simulink model "ES106A_StHlthSigStc"  (R2013b)
settings: Solver=FixedStepDiscrete  SolverMode=SingleTasking  StartTime=0.0  StopTime=1  FixedStep=0.002  RelTol=1e-3
values from neighbouring files (symbols this model uses):
  APPL10_CNT_U08 = DataDict.Constant    [ES106A_StHlthSigStc_DataDict.m]
  BITSPERBYTE_CNT_U08 = DataDict.Constant    [ES106A_StHlthSigStc_DataDict.m]
  ENOTOK_CNT_U08 = DataDict.Constant    [ES106A_StHlthSigStc_DataDict.m]
  EOK_CNT_U08 = DataDict.Constant    [ES106A_StHlthSigStc_DataDict.m]
  LOWRMASKVAL_CNT_U32 = DataDict.Constant    [ES106A_StHlthSigStc_DataDict.m]
  NROFCRCAREA_CNT_U08 = DataDict.ConfigParam    [ES106A_StHlthSigStc_DataDict.m]
  NVMAVRGPOSN_CNT_U08 = DataDict.Constant    [ES106A_StHlthSigStc_DataDict.m]
  NVMMAXPOSN_CNT_U08 = DataDict.Constant    [ES106A_StHlthSigStc_DataDict.m]
  NVMMINPOSN_CNT_U08 = DataDict.Constant    [ES106A_StHlthSigStc_DataDict.m]
  NVMSAMPLECNTRPOSN_CNT_U08 = DataDict.Constant    [ES106A_StHlthSigStc_DataDict.m]
  RAMAVRGPOSN_CNT_U08 = DataDict.Constant    [ES106A_StHlthSigStc_DataDict.m]
  RAMMAXPOSN_CNT_U08 = DataDict.Constant    [ES106A_StHlthSigStc_DataDict.m]
  RAMMINPOSN_CNT_U08 = DataDict.Constant    [ES106A_StHlthSigStc_DataDict.m]
  RAMRAWPOSN_CNT_U08 = DataDict.Constant    [ES106A_StHlthSigStc_DataDict.m]
  SIGCNT_ULS_U08 = DataDict.ConfigParam    [ES106A_StHlthSigStc_DataDict.m]
  SigStcPrmInst = DataDict.PIM    [ES106A_StHlthSigStc_DataDict.m]
  STHLTHMAXVAL_CNT_U08 = DataDict.Constant    [ES106A_StHlthSigStc_DataDict.m]
  WORDSIZE_CNT_U08 = DataDict.Constant    [ES106A_StHlthSigStc_DataDict.m]
undefined symbols (not defined in the file or in its folder): NvmGetErrSts1, StHlthTaskRef1
libraries: simulink x37, NxtrNvM x4, NxtrMax x4, NxtrMin x4
(part 1 of 5)
settings Model: Creator=SumitG  LastModifiedBy=BZHF94
settings SolverCC: AutoInsertRateTranBlk=on  InsertRTBMode=Always
settings DataIOCC: LimitDataPoints=off  SaveFormat=Structure  ReturnWorkspaceOutputs=on
settings OptimizationCC: BlockReduction=off  InlineParams=on  ZeroExternalMemoryAtStartup=off  ZeroInternalMemoryAtStartup=off  OptimizeModelRefInitCode=on  LifeSpan=1
settings DebuggingCC: SignalInfNanChecking=error  SignalRangeChecking=warning  UnderspecifiedInitializationDetection=Simplified  SolverPrmCheckMsg=error  InheritedTsInSrcMsg=error  DiscreteInheritContinuousMsg=error  SingleTaskRateTransMsg=error  TasksWithSamePriorityMsg=error  SigSpecEnsureSampleTimeMsg=error  CheckMatrixSingularityMsg=error  ParameterUnderflowMsg=error  ParameterPrecisionLossMsg=error  ParameterTunabilityLossMsg=error  FixptConstUnderflowMsg=warning  FixptConstOverflowMsg=warning  VectorMatrixConversionMsg=error  SignalLabelMismatchMsg=error  UnconnectedInputMsg=error  UnconnectedOutputMsg=error  UnconnectedLineMsg=error  SFcnCompatibilityMsg=error  UniqueDataStoreMsg=warning  BusObjectLabelMismatch=error  RootOutportRequireBusObject=error  AssertControl=DisableAll  ModelReferenceIOMsg=error  ModelReferenceVersionMismatchMessage=warning  ModelReferenceIOMismatchMessage=error  ModelReferenceCSMismatchMessage=warning  ModelReferenceDataLoggingMessage=error  StateNameClashWarn=warning  StrictBusMsg=ErrorOnBusTreatedAsVector  NonBusSignalsTreatedAsBus=error  SFUnexpectedBacktrackingDiag=error  SFInvalidInputDataAccessInChartInitDiag=error  SFNoUnconditionalDefaultTransitionDiag=error  SFTransitionOutsideNaturalParentDiag=error  SFUnconditionalTransitionShadowingDiag=error  SFUndirectedBroadcastEventsDiag=error
settings ModelReferenceCC: ModelReferenceNumInstancesAllowed=Single
settings RTWCC: SystemTargetFile=autosar.tlc  GenCodeOnly=on  TemplateMakefile=ert_default_tmf  Description=AUTOSAR  GenerateReport=on  ProcessScript=autosar_make_rtw_hook  LaunchReport=on
settings CodeAppCC: GenerateComments=off  IgnoreCustomStorageClasses=off  CustomSymbolStrType=$N$R$M  CustomSymbolStrBlkIO=$N$M  SimulinkBlockComments=off
settings STFCustomTargetCC: ParMdlRefBuildCompliant=on  CompOptLevelCompliant=on  IncludeMdlTerminateFcn=off  CombineOutputUpdateFcns=on  SuppressErrorStatus=on  ERTFirstTimeCompliant=on  ERTCustomFileBanners=on  SupportNonFinite=off  SupportComplex=off  SupportContinuousTime=off  SupportNonInlinedSFcns=off  MATLABClassNameForMDSCustomization=Simulink.SoftwareTarget.ERTCustomization  AutosarCompliant=on  GRTInterface=off  SystemTargetFile=autosar.tlc
settings ERTTargetCC: CodeReplacementLibrary=ANSI_C  ConcurrentExecutionCompliant=off  IncludeMdlTerminateFcn=off  SuppressErrorStatus=on  SupportNonFinite=off  SupportComplex=off  ModelStepFunctionPrototypeControlCompliant=off  CPPClassGenCompliant=off  AutosarCompliant=on  InlinedParameterPlacement=NonHierarchical  ERTCustomFileTemplate=example_file_process.tlc  EnableUserReplacementTypes=on

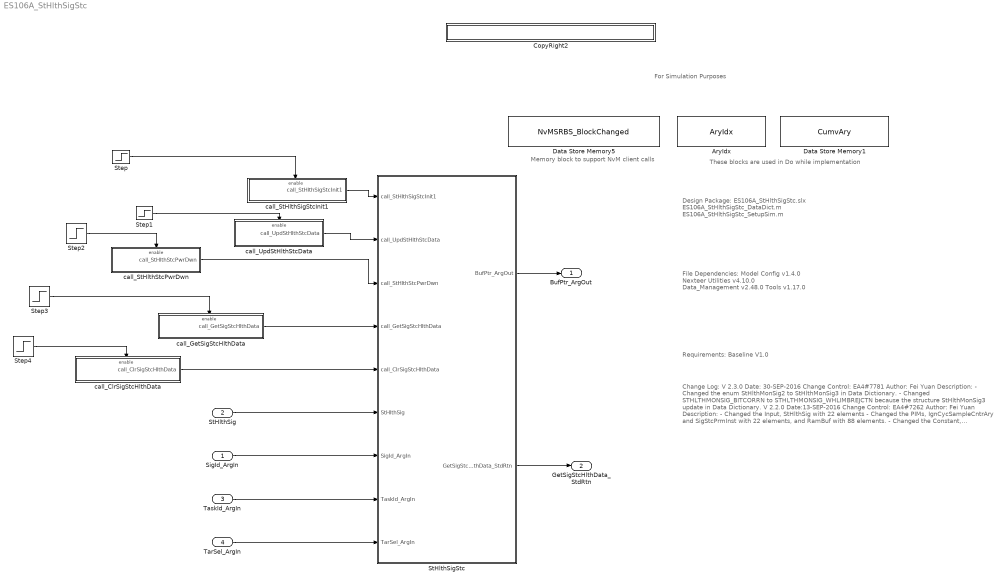
== system ES106A_StHlthSigStc ==
  note: These blocks are used in Do while implementation
  note: For Simulation Purposes
  note: Memory block to support NvM client calls
  note: Requirements: Baseline V1.0
  note: File Dependencies:
      |
      | Model Config v1.4.0
      | Nexteer Utilities v4.10.0
      | Data_Management v2.48.0
      | Tools v1.17.0
  note: Change Log:
      |
      | V 2.3.0
      | Date: 30-SEP-2016
      | Change Control: EA4#7781
      | Author: Fei Yuan
      | Description:
      | - Changed the enum StHlthMonSig2 to StHlthMonSig3 in Data Dictionary.
      | - Changed STHLTHMONSIG_BITCORRN to STHLTHMONSIG_WHLIMBREJCTN because the structure StHlthMonSig3 update in
      |   Data Dictionary.
      |
      | V 2.2.0
      | Date:13-SEP-2016
      | Change Control: EA4#7262
      | Author: Fei Yuan
      | Description:
      | - Changed the Input, StHlthSig with 22 elements
      | - Changed the PIMs, IgnCycSampleCntrAry and SigStcPrmInst with 22 elements, and RamBuf with 88 elements.
      | - Changed the Constant, SIGCNT_ULS_U08.EngVal to 22.
      | - Changed the input port size of the selectors in the model in red.
      |
      | V 2.1.0
      | Date: 2-MAY-2016
      | Change Control:  EA4#5551
      | Author: Sumit Kumar Gupta (KPIT)
      | Description:
      | - Logic added to handle 20 input signals at following subystems:
      | ES106A_StHlthSigStc/StHlthSigStc/StHlthSigStcInit1/For Simulation Purpose
      | ES106A_StHlthSigStc/StHlthSigStc/ClrSigStcHlthData/ClrDataSample/For Iterator Subsystem
      | ES106A_StHlthSigStc/StHlthSigStc/ClrSigStcHlthData/Call Non Trusted Function/For Iterator Subsystem
      |
      | - Due to MIL failures, Ram Buffer and Signal Statistic History Data Array logic is updated at following path:
      | ES106A_StHlthSigStc/StHlthSigStc/UpdStHlthStcData/UpdDataSample/For Iterator Subsystem/Subsystem2/UpdateRamBuf
      | ES106A_StHlthSigStc/StHlthSigStc/UpdStHlthStcData/Call Non Trusted Function /For Iterator Subsystem/Subsystem2/UpdateRamBuf
      | ES106A_StHlthSigStc/StHlthSigStc/StHlthStcPwrDwn/For Iterator Subsystem/If Action Subsystem/Update Nvm
      |
      | V 2.0.0
      | Date: 27-APR-2016
      | Change Control # EA4#5551
      | Author: Sumit Kumar Gupta (KPIT)
      | Description:
      | - Made the changes suggested during MIL and
      | - Changed the design to have 20 input signals coming from ES105A
      |
      | V 1.0.0
      | Date: 11-Feb-2016
      | Change Control # EA4#3078
      | Author: Sumit Kumar Gupta (KPIT)
      | Description:
      | - Initial Release
  note: Design Package:
      |
      | ES106A_StHlthSigStc.slx
      | ES106A_StHlthSigStc_DataDict.m
      | ES106A_StHlthSigStc_SetupSim.m
  SigId_ArgIn : Inport
  StHlthSig : Inport  Port=2  PortDimensions=22
  TaskId_ArgIn : Inport  Port=3
  TarSel_ArgIn : Inport  Port=4
  AryIdx : DataStoreMemory  DataStoreName=AryIdx
  CopyRight2 : Subsystem  Description=|  mask(Copyright Information){none=on}
      | Copyright info block.                                               
      |                                                                     
      | Place copyright information at the top of every subsystem in design.
      mask prompts: none "No parameters"
      mask help: Place copyright information at the top of every subsystem in design.
      mask Display:
      | NxtrConf = 'Nexteer Confidential';
      | 
      | sys = bdroot; %handle for the current model ("system")
      | first = get_param(sys,'Created');
      | if(isempty(first))
      |     first = datestr(now,'yyyy');
      | else
      |     first = first(end-3:end);  %year is last four digits
      | end
      | 
      | last = get_param(sys,'LastModifiedDate');
      | if isempty(last)
      |     last = datestr(now,'yyyy');
      | else
      |     last = last(end-3:end);
      | end
      | 
      | if strcmp(first,last)
      |     fprintf('%s -- Copyright %s Nexteer',NxtrConf,first)
      | else
      |     fprintf('%s -- %s%s- %s Nexteer',NxtrConf,char(169),first,last)
      | end
  Data Store Memory1 : DataStoreMemory  DataStoreName=CumvAry  OutDataTypeStr=uint32
  Data Store Memory5 : DataStoreMemory  DataStoreName=NvMSRBS_BlockChanged
  StHlthSigStc : Subsystem  RequirementInfo={'linktype_rmi_doors' '0001022b (/ESG Group/FDD Module Requirements/EA4 Specific/ES106A_StHlthSigStc )' '#ES106A_5' 'true' 'REQ:ES106A_5' '' ; 'linktype_rmi_doors' '0001022b (/ESG Group/FDD Module Requirements/EA4 Specific/ES106A_StHlthSigStc )' '#ES106A_7' 'true' 'REQ:ES106A_7' '' ; 'linktype_rmi_doors' '0001022b (/ESG Group/FDD Module Requirements/EA4 Specific/ES106A_StHlthSigStc )' '#ES106A_8' 'true' 'REQ:ES106A_8' '' } %GIDa_68933fcf_5356_4a06_a46b_928b692515f7
  Step : Step  Time=0.002  Before=1  After=0  SampleTime=0
  Step1 : Step  Time=0.002  SampleTime=0
  Step2 : Step  Time=0.25  SampleTime=0
  Step3 : Step  Time=0.006  SampleTime=0
  Step4 : Step  Time=0.006  SampleTime=0
  call_ClrSigStcHlthData : Subsystem  TreatAsAtomicUnit=on
  call_GetSigStcHlthData : Subsystem  TreatAsAtomicUnit=on
  call_StHlthSigStcInit1 : Subsystem  TreatAsAtomicUnit=on
  call_StHlthStcPwrDwn : Subsystem  TreatAsAtomicUnit=on
  call_UpdStHlthStcData : Subsystem  TreatAsAtomicUnit=on
  BufPtr_ArgOut : Outport
  GetSigStcHlthData_StdRtn : Outport  Port=2
  wires:
  call_StHlthSigStcInit1/1(call_StHlthSigStcInit1) -> StHlthSigStc/1(call_StHlthSigStcInit1)
  call_UpdStHlthStcData/1(call_UpdStHlthStcData) -> StHlthSigStc/2(call_UpdStHlthStcData)
  Step1/1 -> call_UpdStHlthStcData/Enable
  Step/1 -> call_StHlthSigStcInit1/Enable
  Step2/1 -> call_StHlthStcPwrDwn/Enable
  Step3/1 -> call_GetSigStcHlthData/Enable
  StHlthSigStc/1(BufPtr_ArgOut) -> BufPtr_ArgOut/1
  Step4/1 -> call_ClrSigStcHlthData/Enable
  call_StHlthStcPwrDwn/1(call_StHlthStcPwrDwn) -> StHlthSigStc/3(call_StHlthStcPwrDwn)
  call_GetSigStcHlthData/1(call_GetSigStcHlthData) -> StHlthSigStc/4(call_GetSigStcHlthData)
  call_ClrSigStcHlthData/1(call_ClrSigStcHlthData) -> StHlthSigStc/5(call_ClrSigStcHlthData)
  SigId_ArgIn/1 -> StHlthSigStc/7(SigId_ArgIn)
  StHlthSig/1 -> StHlthSigStc/6(StHlthSig)
  TaskId_ArgIn/1 -> StHlthSigStc/8(TaskId_ArgIn)
  TarSel_ArgIn/1 -> StHlthSigStc/9(TarSel_ArgIn)
  StHlthSigStc/2(GetSigStcHlthData_StdRtn) -> GetSigStcHlthData_StdRtn/1

== system ES106A_StHlthSigStc/CopyRight2 ==

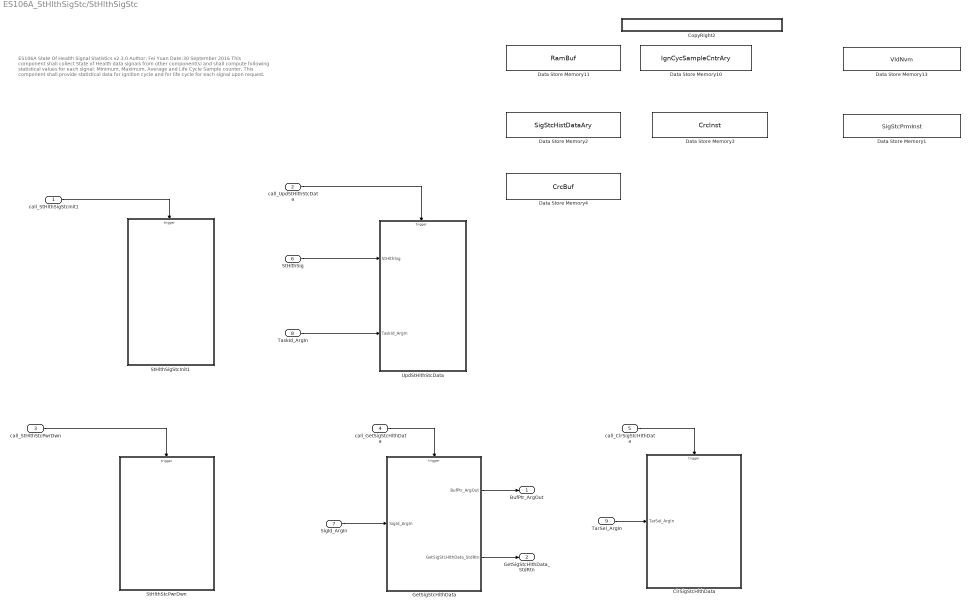
== system ES106A_StHlthSigStc/StHlthSigStc ==
  note: ES106A  State Of Health Signal Statistics
      | v2.3.0 								 Author: Fei Yuan                                                                               Date:30 September 2016
      |
      |   This component shall collect State of Health data signals from other component(s) and shall compute following statistical values for each
      |   signal: Minimum, Maximum, Average and Life Cycle Sample counter. This component shall provide statistical data for ignition cycle and
      |   for life cycle for each signal upon request.
  call_StHlthSigStcInit1 : Inport
  call_UpdStHlthStcData : Inport  Port=2
  call_StHlthStcPwrDwn : Inport  Port=3
  call_GetSigStcHlthData : Inport  Port=4
  call_ClrSigStcHlthData : Inport  Port=5
  StHlthSig : Inport  RequirementInfo={'linktype_rmi_doors' '0001022b (/ESG Group/FDD Module Requirements/EA4 Specific/ES106A_StHlthSigStc )' '#ES106A_6' 'true' 'REQ:ES106A_6' '' } %GIDa_de3f5b39_a288_4714_b61d_c77c2ab3aa56  Port=6
  SigId_ArgIn : Inport  Port=7
  TaskId_ArgIn : Inport  Port=8
  TarSel_ArgIn : Inport  Port=9
  ClrSigStcHlthData : Subsystem  RequirementInfo={'linktype_rmi_doors' '0001022b (/ESG Group/FDD Module Requirements/EA4 Specific/ES106A_StHlthSigStc )' '#ES106A_39' 'true' 'REQ:ES106A_39' '' ; 'linktype_rmi_doors' '0001022b (/ESG Group/FDD Module Requirements/EA4 Specific/ES106A_StHlthSigStc )' '#ES106A_40' 'true' 'REQ:ES106A_40' '' } %GIDa_0e6a92ad_9a1d_4662_a746_e45f4d082b4b  TreatAsAtomicUnit=on
  CopyRight2 : Subsystem  Description=|  mask(Copyright Information){none=on}
      | Copyright info block.                                               
      |                                                                     
      | Place copyright information at the top of every subsystem in design.
      mask prompts: none "No parameters"
      mask help: Place copyright information at the top of every subsystem in design.
      mask Display:
      | NxtrConf = 'Nexteer Confidential';
      | 
      | sys = bdroot; %handle for the current model ("system")
      | first = get_param(sys,'Created');
      | first = first(end-3:end);  %year is last four digits
      | 
      | last = get_param(sys,'LastModifiedDate');
      | if isempty(last)
      |     last = datestr(now,'yyyy');
      | else
      |     last = last(end-3:end);
      | end
      | 
      | if strcmp(first,last)
      |     fprintf('%s -- Copyright %s Nexteer',NxtrConf,first)
      | else
      |     fprintf('%s -- %s%s- %s Nexteer',NxtrConf,char(169),first,last)
      | end
  Data Store Memory1 : DataStoreMemory  Description=|  DataStoreName=SigStcPrmInst  InitialValue=[0 0 0 0 0 0 0 0 0 0 0 0 0 0 0 0 0 0 0 0 0 0]  OutDataTypeStr=Bus: StHlthSigStcPrmRec1
      | Length is a ConfigParam in STHLTHSIGSTCSIGCNT_ULS_U08.
      | This is the configurable macro. This is generated out of DaVinci Configurator.
      | As an example for simulation purpose, we have 2 elements which contain detials about EcuT & Voltage.
      settings: AttributesFormatString=%<Description>
  Data Store Memory10 : DataStoreMemory  Description=|  DataStoreName=IgnCycSampleCntrAry  InitialValue=[]  StateMustResolveToSignalObject=on
      | Maintains number of samples
      | monitored in the present ignition 
      | cycle for every signal
      settings: AttributesFormatString=%<Description>
  Data Store Memory11 : DataStoreMemory  Description=|  DataStoreName=RamBuf  InitialValue=[]  StateMustResolveToSignalObject=on
      | Maintains current sample and statistical 
      | data for current ignition 
      | cycle for every signal
      settings: AttributesFormatString=%<Description>
  Data Store Memory13 : DataStoreMemory  Description=Maintains validity / applicablility of NVM block  DataStoreName=VldNvm  InitialValue=[]  StateMustResolveToSignalObject=on
      settings: AttributesFormatString=%<Description>
  Data Store Memory2 : DataStoreMemory  Description=|  DataStoreName=SigStcHistDataAry  InitialValue=[]  StateMustResolveToSignalObject=on
      | Array containing Min, Max, Avg and 
      | counter values  for all the State of 
      | Health Signals that need to be stored 
      | in NVM
      settings: AttributesFormatString=%<Description>
  Data Store Memory3 : DataStoreMemory  Description=|  DataStoreName=CrcInst  WriteAfterWriteMsg=warning  InitialValue=[0 0 0 0 0 0 0 0]  StateMustResolveToSignalObject=on
      | This a Software configurable generated out of DaVinci Configurator. 
      | As an example for simulation purpose, PIM is used with 2 elements which 
      | contain detials about EcuT and Voltage signals.
      settings: AttributesFormatString=%<Description>
  Data Store Memory4 : DataStoreMemory  Description=|  DataStoreName=CrcBuf  InitialValue=[0 0 0 0 0 0 0 0 0 0 0 0 0 0 0 0 0 0 0 0 0 0 0 0 0 0 0 0 0 0 0 0]
      | This is a local buffer responsible to hold the CRC values for the
      | state health signals.
      settings: AttributesFormatString=%<Description>
  GetSigStcHlthData : Subsystem  RequirementInfo={'linktype_rmi_doors' '0001022b (/ESG Group/FDD Module Requirements/EA4 Specific/ES106A_StHlthSigStc )' '#ES106A_37' 'true' 'REQ:ES106A_37' '' } %GIDa_7dc2dad3_2246_4e59_ab75_d3cb8790f602  TreatAsAtomicUnit=on
  StHlthSigStcInit1 : Subsystem  TreatAsAtomicUnit=on
  StHlthStcPwrDwn : Subsystem  RequirementInfo={'linktype_rmi_doors' '0001022b (/ESG Group/FDD Module Requirements/EA4 Specific/ES106A_StHlthSigStc )' '#ES106A_12' 'true' 'REQ:ES106A_12' '' } %GIDa_956d3843_84ba_4f6a_837a_1be91f390343  TreatAsAtomicUnit=on
  UpdStHlthStcData : Subsystem  RequirementInfo={'linktype_rmi_doors' '0001022b (/ESG Group/FDD Module Requirements/EA4 Specific/ES106A_StHlthSigStc )' '#ES106A_11' 'true' 'REQ:ES106A_11' '' ; 'linktype_rmi_doors' '0001022b (/ESG Group/FDD Module Requirements/EA4 Specific/ES106A_StHlthSigStc )' '#ES106A_35' 'true' 'REQ:ES106A_35' '' } %GIDa_ed89dcf0_9167_4ec8_9b6c_073f14f3c033  TreatAsAtomicUnit=on
  BufPtr_ArgOut : Outport
  GetSigStcHlthData_StdRtn : Outport  Port=2
  wires:
  call_StHlthSigStcInit1/1 -> StHlthSigStcInit1/Trigger
  call_UpdStHlthStcData/1 -> UpdStHlthStcData/Trigger
  call_StHlthStcPwrDwn/1 -> StHlthStcPwrDwn/Trigger
  call_GetSigStcHlthData/1 -> GetSigStcHlthData/Trigger
  GetSigStcHlthData/1(BufPtr_ArgOut) -> BufPtr_ArgOut/1
  SigId_ArgIn/1 -> GetSigStcHlthData/1(SigId_ArgIn)
  call_ClrSigStcHlthData/1 -> ClrSigStcHlthData/Trigger
  GetSigStcHlthData/2(GetSigStcHlthData_StdRtn) -> GetSigStcHlthData_StdRtn/1
  TarSel_ArgIn/1 -> ClrSigStcHlthData/1(TarSel_ArgIn)
  StHlthSig/1 -> UpdStHlthStcData/1(StHlthSig)
  TaskId_ArgIn/1 -> UpdStHlthStcData/2(TaskId_ArgIn)

== system ES106A_StHlthSigStc/call_ClrSigStcHlthData ==
  Enable : EnablePort
  CopyRight2 : Subsystem  Description=|  mask(Copyright Information){none=on}
      | Copyright info block.                                               
      |                                                                     
      | Place copyright information at the top of every subsystem in design.
      mask prompts: none "No parameters"
      mask help: Place copyright information at the top of every subsystem in design.
      mask Display:
      | NxtrConf = 'Nexteer Confidential';
      | 
      | sys = bdroot; %handle for the current model ("system")
      | first = get_param(sys,'Created');
      | if(isempty(first))
      |     first = datestr(now,'yyyy');
      | else
      |     first = first(end-3:end);  %year is last four digits
      | end
      | 
      | last = get_param(sys,'LastModifiedDate');
      | if isempty(last)
      |     last = datestr(now,'yyyy');
      | else
      |     last = last(end-3:end);
      | end
      | 
      | if strcmp(first,last)
      |     fprintf('%s -- Copyright %s Nexteer',NxtrConf,first)
      | else
      |     fprintf('%s -- %s%s- %s Nexteer',NxtrConf,char(169),first,last)
      | end
  Function-Call Generator : simulink/Ports & Subsystems/Function-Call Generator  sample_time=0.002  numberOfIterations=1
  call_ClrSigStcHlthData : Outport
  wires:
  Function-Call Generator/1 -> call_ClrSigStcHlthData/1

== system ES106A_StHlthSigStc/call_GetSigStcHlthData ==
  Enable : EnablePort
  CopyRight2 : Subsystem  Description=|  mask(Copyright Information){none=on}
      | Copyright info block.                                               
      |                                                                     
      | Place copyright information at the top of every subsystem in design.
      mask prompts: none "No parameters"
      mask help: Place copyright information at the top of every subsystem in design.
      mask Display:
      | NxtrConf = 'Nexteer Confidential';
      | 
      | sys = bdroot; %handle for the current model ("system")
      | first = get_param(sys,'Created');
      | if(isempty(first))
      |     first = datestr(now,'yyyy');
      | else
      |     first = first(end-3:end);  %year is last four digits
      | end
      | 
      | last = get_param(sys,'LastModifiedDate');
      | if isempty(last)
      |     last = datestr(now,'yyyy');
      | else
      |     last = last(end-3:end);
      | end
      | 
      | if strcmp(first,last)
      |     fprintf('%s -- Copyright %s Nexteer',NxtrConf,first)
      | else
      |     fprintf('%s -- %s%s- %s Nexteer',NxtrConf,char(169),first,last)
      | end
  Function-Call Generator : simulink/Ports & Subsystems/Function-Call Generator  sample_time=0.002  numberOfIterations=1
  call_GetSigStcHlthData : Outport
  wires:
  Function-Call Generator/1 -> call_GetSigStcHlthData/1

== system ES106A_StHlthSigStc/call_StHlthSigStcInit1 ==
  Enable : EnablePort
  CopyRight2 : Subsystem  Description=|  mask(Copyright Information){none=on}
      | Copyright info block.                                               
      |                                                                     
      | Place copyright information at the top of every subsystem in design.
      mask prompts: none "No parameters"
      mask help: Place copyright information at the top of every subsystem in design.
      mask Display:
      | NxtrConf = 'Nexteer Confidential';
      | 
      | sys = bdroot; %handle for the current model ("system")
      | first = get_param(sys,'Created');
      | first = first(end-3:end);  %year is last four digits
      | 
      | last = get_param(sys,'LastModifiedDate');
      | if isempty(last)
      |     last = datestr(now,'yyyy');
      | else
      |     last = last(end-3:end);
      | end
      | 
      | if strcmp(first,last)
      |     fprintf('%s -- Copyright %s Nexteer',NxtrConf,first)
      | else
      |     fprintf('%s -- %s%s- %s Nexteer',NxtrConf,char(169),first,last)
      | end
  "Function-Call Generator " : simulink/Ports & Subsystems/Function-Call Generator  sample_time=0  numberOfIterations=1
  call_StHlthSigStcInit1 : Outport
  wires:
  "Function-Call Generator "/1 -> call_StHlthSigStcInit1/1

== system ES106A_StHlthSigStc/call_StHlthStcPwrDwn ==
  Enable : EnablePort
  CopyRight2 : Subsystem  Description=|  mask(Copyright Information){none=on}
      | Copyright info block.                                               
      |                                                                     
      | Place copyright information at the top of every subsystem in design.
      mask prompts: none "No parameters"
      mask help: Place copyright information at the top of every subsystem in design.
      mask Display:
      | NxtrConf = 'Nexteer Confidential';
      | 
      | sys = bdroot; %handle for the current model ("system")
      | first = get_param(sys,'Created');
      | if(isempty(first))
      |     first = datestr(now,'yyyy');
      | else
      |     first = first(end-3:end);  %year is last four digits
      | end
      | 
      | last = get_param(sys,'LastModifiedDate');
      | if isempty(last)
      |     last = datestr(now,'yyyy');
      | else
      |     last = last(end-3:end);
      | end
      | 
      | if strcmp(first,last)
      |     fprintf('%s -- Copyright %s Nexteer',NxtrConf,first)
      | else
      |     fprintf('%s -- %s%s- %s Nexteer',NxtrConf,char(169),first,last)
      | end
  Function-Call Generator1 : simulink/Ports & Subsystems/Function-Call Generator  sample_time=0.002  numberOfIterations=1
  call_StHlthStcPwrDwn : Outport
  wires:
  Function-Call Generator1/1 -> call_StHlthStcPwrDwn/1

== system ES106A_StHlthSigStc/call_UpdStHlthStcData ==
  Enable : EnablePort
  CopyRight2 : Subsystem  Description=|  mask(Copyright Information){none=on}
      | Copyright info block.                                               
      |                                                                     
      | Place copyright information at the top of every subsystem in design.
      mask prompts: none "No parameters"
      mask help: Place copyright information at the top of every subsystem in design.
      mask Display:
      | NxtrConf = 'Nexteer Confidential';
      | 
      | sys = bdroot; %handle for the current model ("system")
      | first = get_param(sys,'Created');
      | first = first(end-3:end);  %year is last four digits
      | 
      | last = get_param(sys,'LastModifiedDate');
      | if isempty(last)
      |     last = datestr(now,'yyyy');
      | else
      |     last = last(end-3:end);
      | end
      | 
      | if strcmp(first,last)
      |     fprintf('%s -- Copyright %s Nexteer',NxtrConf,first)
      | else
      |     fprintf('%s -- %s%s- %s Nexteer',NxtrConf,char(169),first,last)
      | end
  "Function-Call Generator " : simulink/Ports & Subsystems/Function-Call Generator  sample_time=0  numberOfIterations=1
  call_UpdStHlthStcData : Outport
  wires:
  "Function-Call Generator "/1 -> call_UpdStHlthStcData/1

== system ES106A_StHlthSigStc/StHlthSigStc/ClrSigStcHlthData ==
  TarSel_ArgIn : Inport
  function : TriggerPort  TriggerType=function-call
  Call Non Trusted Function : Subsystem  TreatAsAtomicUnit=on
  ClrDataSample : Subsystem  TreatAsAtomicUnit=on
  Constant : Constant  Value=APPL10_CNT_U08
  CopyRight2 : Subsystem  Description=|  mask(Copyright Information){none=on}
      | Copyright info block.                                               
      |                                                                     
      | Place copyright information at the top of every subsystem in design.
      mask prompts: none "No parameters"
      mask help: Place copyright information at the top of every subsystem in design.
      mask Display:
      | NxtrConf = 'Nexteer Confidential';
      | 
      | sys = bdroot; %handle for the current model ("system")
      | first = get_param(sys,'Created');
      | first = first(end-3:end);  %year is last four digits
      | 
      | last = get_param(sys,'LastModifiedDate');
      | if isempty(last)
      |     last = datestr(now,'yyyy');
      | else
      |     last = last(end-3:end);
      | end
      | 
      | if strcmp(first,last)
      |     fprintf('%s -- Copyright %s Nexteer',NxtrConf,first)
      | else
      |     fprintf('%s -- %s%s- %s Nexteer',NxtrConf,char(169),first,last)
      | end
  GetApplicationID : Subsystem
  If : If  IfExpression=u1
  Relational Operator : RelationalOperator  Operator===  OutDataTypeStr=boolean
  wires:
  TarSel_ArgIn/1 -> Call Non Trusted Function/1(TarSel_ArgIn), ClrDataSample/1(TarSel_ArgIn)
  If/1 -> ClrDataSample/Action
  If/2 -> Call Non Trusted Function/Action
  GetApplicationID/1(ApplId) -> Relational Operator/1
  Constant/1 -> Relational Operator/2
  Relational Operator/1 -> If/1

== system ES106A_StHlthSigStc/StHlthSigStc/CopyRight2 ==

== system ES106A_StHlthSigStc/StHlthSigStc/GetSigStcHlthData ==
  SigId_ArgIn : Inport
  function : TriggerPort  TriggerType=function-call
  Constant : Constant  Value=SIGCNT_ULS_U08
  CopyRight2 : Subsystem  Description=|  mask(Copyright Information){none=on}
      | Copyright info block.                                               
      |                                                                     
      | Place copyright information at the top of every subsystem in design.
      mask prompts: none "No parameters"
      mask help: Place copyright information at the top of every subsystem in design.
      mask Display:
      | NxtrConf = 'Nexteer Confidential';
      | 
      | sys = bdroot; %handle for the current model ("system")
      | first = get_param(sys,'Created');
      | first = first(end-3:end);  %year is last four digits
      | 
      | last = get_param(sys,'LastModifiedDate');
      | if isempty(last)
      |     last = datestr(now,'yyyy');
      | else
      |     last = last(end-3:end);
      | end
      | 
      | if strcmp(first,last)
      |     fprintf('%s -- Copyright %s Nexteer',NxtrConf,first)
      | else
      |     fprintf('%s -- %s%s- %s Nexteer',NxtrConf,char(169),first,last)
      | end
  If : If  IfExpression=u1
  If Action Subsystem : Subsystem  TreatAsAtomicUnit=on
  If Action Subsystem1 : Subsystem  TreatAsAtomicUnit=on
  Merge : Merge
  Relational Operator : RelationalOperator  Operator=<  OutDataTypeStr=boolean
  BufPtr_ArgOut : Outport
  GetSigStcHlthData_StdRtn : Outport  Port=2
  wires:
  SigId_ArgIn/1 -> If Action Subsystem1/1(In1), Relational Operator/1
  Relational Operator/1 -> If/1
  If/2 -> If Action Subsystem/Action
  If/1 -> If Action Subsystem1/Action
  If Action Subsystem/1(GetSigStcHlthData_StdRtn) -> Merge/2
  If Action Subsystem1/1(BufPtr_ArgOut) -> BufPtr_ArgOut/1
  If Action Subsystem1/2(GetSigStcHlthData_StdRtn) -> Merge/1
  Merge/1 -> GetSigStcHlthData_StdRtn/1
  Constant/1 -> Relational Operator/2

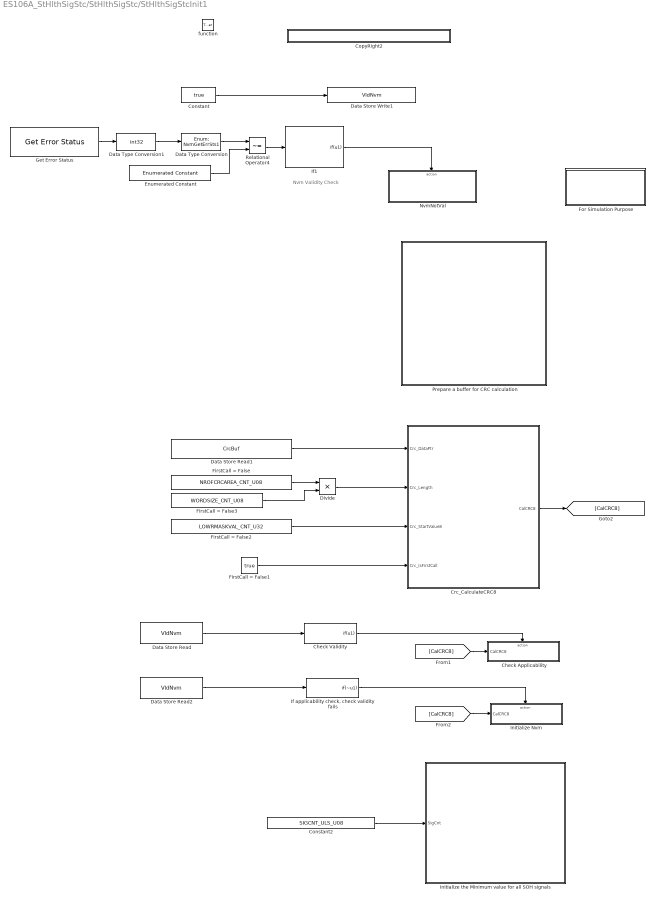
== system ES106A_StHlthSigStc/StHlthSigStc/StHlthSigStcInit1 ==
  note: Nvm Validity Check
  function : TriggerPort  TriggerType=function-call
  Check Applicability : Subsystem  RequirementInfo={'linktype_rmi_doors' '0001022b (/ESG Group/FDD Module Requirements/EA4 Specific/ES106A_StHlthSigStc )' '#ES106A_43' 'true' 'REQ:ES106A_43' '' } %GIDa_cf1830ec_5f38_44f0_b2bb_faccdd1dab0d  TreatAsAtomicUnit=on
  Check Validity : If  RequirementInfo={'linktype_rmi_doors' '0001022b (/ESG Group/FDD Module Requirements/EA4 Specific/ES106A_StHlthSigStc )' '#ES106A_43' 'true' 'REQ:ES106A_43' '' } %GIDa_b8348bd8_3140_476f_ba35_06d587dfd308  IfExpression=u1  ShowElse=off
  Constant : Constant  Value=true  OutDataTypeStr=boolean
      settings: AttributesFormatString=%<OutDataTypeStr>
  Constant2 : Constant  Value=SIGCNT_ULS_U08
  CopyRight2 : Subsystem  Description=|  mask(Copyright Information){none=on}
      | Copyright info block.                                               
      |                                                                     
      | Place copyright information at the top of every subsystem in design.
      mask prompts: none "No parameters"
      mask help: Place copyright information at the top of every subsystem in design.
      mask Display:
      | NxtrConf = 'Nexteer Confidential';
      | 
      | sys = bdroot; %handle for the current model ("system")
      | first = get_param(sys,'Created');
      | first = first(end-3:end);  %year is last four digits
      | 
      | last = get_param(sys,'LastModifiedDate');
      | if isempty(last)
      |     last = datestr(now,'yyyy');
      | else
      |     last = last(end-3:end);
      | end
      | 
      | if strcmp(first,last)
      |     fprintf('%s -- Copyright %s Nexteer',NxtrConf,first)
      | else
      |     fprintf('%s -- %s%s- %s Nexteer',NxtrConf,char(169),first,last)
      | end
  Crc_CalculateCRC8 : Subsystem  RequirementInfo={'linktype_rmi_doors' '0001022b (/ESG Group/FDD Module Requirements/EA4 Specific/ES106A_StHlthSigStc )' '#ES106A_49' 'true' 'REQ:ES106A_49' '' } %GIDa_fe7260c2_c5d7_4f68_aa17_7c606eb91c89
  Data Store Read : DataStoreRead  DataStoreName=VldNvm
  Data Store Read1 : DataStoreRead  DataStoreName=CrcBuf
  Data Store Read2 : DataStoreRead  DataStoreName=VldNvm
  Data Store Write1 : DataStoreWrite  DataStoreName=VldNvm
  Data Type Conversion : DataTypeConversion  RequirementInfo={} %GIDa_f3c2567b_ce70_431c_9ab0_fa5b8c68088e  OutDataTypeStr=Enum: NvmGetErrSts1
  Data Type Conversion1 : DataTypeConversion  RequirementInfo={} %GIDa_3557f0c9_4441_4a2e_8d97_8350f52e6630  OutDataTypeStr=int32
  Divide : Product  Inputs=**
  Enumerated Constant : simulink/Sources/Enumerated Constant  RequirementInfo={'linktype_rmi_doors' '0001022b (/ESG Group/FDD Module Requirements/EA4 Specific/ES106A_StHlthSigStc )' '#ES106A_53' 'true' 'REQ:ES106A_53' '' } %GIDa_54684be9_3785_4eb9_846e_3abfb5e597d9  OutDataTypeStr=Enum: NvmGetErrSts1  Value=NvmGetErrSts1.REQUEST_OK  SampleTime=inf
  FirstCall = False : Constant  Value=NROFCRCAREA_CNT_U08
  FirstCall = False1 : Constant  Value=true  OutDataTypeStr=boolean
      settings: AttributesFormatString=%<OutDataTypeStr>
  FirstCall = False2 : Constant  Value=LOWRMASKVAL_CNT_U32
  FirstCall = False3 : Constant  Value=WORDSIZE_CNT_U08
  For Simulation Purpose : Subsystem
  Get Error Status : NxtrNvM/Get Error Status  RequirementInfo={'linktype_rmi_doors' '0001022b (/ESG Group/FDD Module Requirements/EA4 Specific/ES106A_StHlthSigStc )' '#ES106A_52' 'true' 'REQ:ES106A_52' '' ; 'linktype_rmi_doors' '0001022b (/ESG Group/FDD Module Requirements/EA4 Specific/ES106A_StHlthSigStc )' '#ES106A_53' 'true' 'REQ:ES106A_53' '' } %GIDa_399198bd_5409_4802_827c_472582b442de  FuncName=Get Error Status  NvMBlockName=SigStcHistDataAry  VoidFuncRtn=on  ReqResPtr_DSN=NvMGES_ReqResPtr  Return_DSN=NvMGES_ReqResPtr
      settings: AttributesFormatString=%<FuncName>
  "If applicability check, check validity fails" : If  RequirementInfo={'linktype_rmi_doors' '0001022b (/ESG Group/FDD Module Requirements/EA4 Specific/ES106A_StHlthSigStc )' '#ES106A_43' 'true' 'REQ:ES106A_43' '' } %GIDa_476b5806_828d_4d52_b3b9_6820ae4d778b  IfExpression=~u1  ShowElse=off
  If1 : If  RequirementInfo={'linktype_rmi_doors' '0001022b (/ESG Group/FDD Module Requirements/EA4 Specific/ES106A_StHlthSigStc )' '#ES106A_52' 'true' 'REQ:ES106A_52' '' } %GIDa_9637d3dc_c7d4_43ae_a1cc_bc1496dec7e3  Priority=0  IfExpression=u1  ShowElse=off
  Initialize Nvm : Subsystem  RequirementInfo={'linktype_rmi_doors' '0001022b (/ESG Group/FDD Module Requirements/EA4 Specific/ES106A_StHlthSigStc )' '#ES106A_44' 'true' 'REQ:ES106A_44' '' } %GIDa_6928d7f4_7d67_425e_af74_57ec55e9a845  TreatAsAtomicUnit=on
  Initialize the Minimum value for all SOH signals : Subsystem  RequirementInfo={'linktype_rmi_doors' '0001022b (/ESG Group/FDD Module Requirements/EA4 Specific/ES106A_StHlthSigStc )' '#ES106A_14' 'true' 'REQ:ES106A_14' '' ; 'linktype_rmi_doors' '0001022b (/ESG Group/FDD Module Requirements/EA4 Specific/ES106A_StHlthSigStc )' '#ES106A_17' 'true' 'REQ:ES106A_17' '' ; 'linktype_rmi_doors' '0001022b (/ESG Group/FDD Module Requirements/EA4 Specific/ES106A_StHlthSigStc )' '#ES106A_20' 'true' 'REQ:ES106A_20' '' } %GIDa_4ea75232_ebdd_44c0_a5fa_f3833cddec7a  TreatAsAtomicUnit=on
  NvmNotVal : Subsystem  RequirementInfo={'linktype_rmi_doors' '0001022b (/ESG Group/FDD Module Requirements/EA4 Specific/ES106A_StHlthSigStc )' '#ES106A_43' 'true' 'REQ:ES106A_43' '' ; 'linktype_rmi_doors' '0001022b (/ESG Group/FDD Module Requirements/EA4 Specific/ES106A_StHlthSigStc )' '#ES106A_54' 'true' 'REQ:ES106A_54' '' } %GIDa_e952b128_a58e_45a9_9ef5_e77a87821c7b  TreatAsAtomicUnit=on
  Prepare a buffer for CRC calculation : Subsystem  TreatAsAtomicUnit=on
  Relational Operator4 : RelationalOperator  RequirementInfo={'linktype_rmi_doors' '0001022b (/ESG Group/FDD Module Requirements/EA4 Specific/ES106A_StHlthSigStc )' '#ES106A_52' 'true' 'REQ:ES106A_52' '' } %GIDa_b4b3c802_dd5e_49c5_9a14_91cdc6cb1bba  Operator=~=  OutDataTypeStr=boolean
  wires:
  If1/1 -> NvmNotVal/Action
  Relational Operator4/1 -> If1/1
  Enumerated Constant/1 -> Relational Operator4/2
  Data Type Conversion/1 -> Relational Operator4/1
  Get Error Status/1 -> Data Type Conversion1/1
  Data Store Read/1 -> Check Validity/1
  Check Validity/1 -> Check Applicability/Action
  FirstCall = False/1 -> Divide/1
  FirstCall = False1/1 -> Crc_CalculateCRC8/4(Crc_IsFirstCall)
  FirstCall = False2/1 -> Crc_CalculateCRC8/3(Crc_StartValue8)
  FirstCall = False3/1 -> Divide/2
  Crc_CalculateCRC8/1(CalCRC8) -> [CalCRC8]
  [CalCRC8] -> Check Applicability/1(CalCRC8)
  [CalCRC8] -> Initialize Nvm/1(CalCRC8)
  Divide/1 -> Crc_CalculateCRC8/2(Crc_Length)
  Constant2/1 -> Initialize the Minimum value for all SOH signals/1(SigCnt)
  Data Store Read1/1 -> Crc_CalculateCRC8/1(Crc_DataPtr)
  Constant/1 -> Data Store Write1/1
  Data Store Read2/1 -> "If applicability check, check validity fails"/1
  "If applicability check, check validity fails"/1 -> Initialize Nvm/Action
  Data Type Conversion1/1 -> Data Type Conversion/1

== system ES106A_StHlthSigStc/StHlthSigStc/StHlthStcPwrDwn ==
  function : TriggerPort  TriggerType=function-call
  Constant1 : Constant  Value=SIGCNT_ULS_U08
  CopyRight2 : Subsystem  Description=|  mask(Copyright Information){none=on}
      | Copyright info block.                                               
      |                                                                     
      | Place copyright information at the top of every subsystem in design.
      mask prompts: none "No parameters"
      mask help: Place copyright information at the top of every subsystem in design.
      mask Display:
      | NxtrConf = 'Nexteer Confidential';
      | 
      | sys = bdroot; %handle for the current model ("system")
      | first = get_param(sys,'Created');
      | first = first(end-3:end);  %year is last four digits
      | 
      | last = get_param(sys,'LastModifiedDate');
      | if isempty(last)
      |     last = datestr(now,'yyyy');
      | else
      |     last = last(end-3:end);
      | end
      | 
      | if strcmp(first,last)
      |     fprintf('%s -- Copyright %s Nexteer',NxtrConf,first)
      | else
      |     fprintf('%s -- %s%s- %s Nexteer',NxtrConf,char(169),first,last)
      | end
  For Iterator Subsystem : Subsystem  TreatAsAtomicUnit=on
  wires:
  Constant1/1 -> For Iterator Subsystem/1(SigCnt)

== system ES106A_StHlthSigStc/StHlthSigStc/UpdStHlthStcData ==
  StHlthSig : Inport
  TaskId_ArgIn : Inport  Port=2
  function : TriggerPort  TriggerType=function-call
  "Call Non Trusted Function " : Subsystem  TreatAsAtomicUnit=on
  Constant : Constant  RequirementInfo="{}  %GIDa_98965ea7_070e_4143_8e57_1d60cf85e379"  Value=SIGCNT_ULS_U08  OutDataTypeStr=uint8
      settings: AttributesFormatString=%<OutDataTypeStr>
  Constant1 : Constant  Value=APPL10_CNT_U08
  CopyRight2 : Subsystem  Description=|  mask(Copyright Information){none=on}
      | Copyright info block.                                               
      |                                                                     
      | Place copyright information at the top of every subsystem in design.
      mask prompts: none "No parameters"
      mask help: Place copyright information at the top of every subsystem in design.
      mask Display:
      | NxtrConf = 'Nexteer Confidential';
      | 
      | sys = bdroot; %handle for the current model ("system")
      | first = get_param(sys,'Created');
      | first = first(end-3:end);  %year is last four digits
      | 
      | last = get_param(sys,'LastModifiedDate');
      | if isempty(last)
      |     last = datestr(now,'yyyy');
      | else
      |     last = last(end-3:end);
      | end
      | 
      | if strcmp(first,last)
      |     fprintf('%s -- Copyright %s Nexteer',NxtrConf,first)
      | else
      |     fprintf('%s -- %s%s- %s Nexteer',NxtrConf,char(169),first,last)
      | end
  GetApplicationID : Subsystem
  If : If  IfExpression=u1
  Relational Operator : RelationalOperator  Operator===  OutDataTypeStr=boolean
  UpdDataSample : Subsystem  TreatAsAtomicUnit=on
  wires:
  If/1 -> UpdDataSample/Action
  If/2 -> "Call Non Trusted Function "/Action
  GetApplicationID/1(ApplId) -> Relational Operator/1
  Constant1/1 -> Relational Operator/2
  Relational Operator/1 -> If/1
  TaskId_ArgIn/1 -> "Call Non Trusted Function "/2(TaskId_ArgIn), UpdDataSample/2(TaskId_ArgIn)
  StHlthSig/1 -> "Call Non Trusted Function "/1(StHlthSig), UpdDataSample/1(StHlthSig)
  Constant/1 -> "Call Non Trusted Function "/3(SigCnt), UpdDataSample/3(SigCnt)

== system ES106A_StHlthSigStc/call_ClrSigStcHlthData/CopyRight2 ==

== system ES106A_StHlthSigStc/call_GetSigStcHlthData/CopyRight2 ==

== system ES106A_StHlthSigStc/call_StHlthSigStcInit1/CopyRight2 ==

== system ES106A_StHlthSigStc/call_StHlthStcPwrDwn/CopyRight2 ==

== system ES106A_StHlthSigStc/call_UpdStHlthStcData/CopyRight2 ==

== system ES106A_StHlthSigStc/StHlthSigStc/ClrSigStcHlthData/Call Non Trusted Function ==
  TarSel_ArgIn : Inport
  Action Port : ActionPort  ActionType=else
  Assignment1 : Assignment  IndexMode=Zero-based  IndexOptions=Assign all  Indices=1  OutputSizes=1
  Assignment4 : Assignment  IndexMode=Zero-based  IndexOptions=Assign all  Indices=1  OutputSizes=1
  Clear Nvm Data : Subsystem  TreatAsAtomicUnit=on
  Constant : Constant  Value=SIGCNT_ULS_U08
  Constant1 : Constant  Value=0  OutDataTypeStr=uint8
  Constant4 : Constant  Value=0  OutDataTypeStr=uint32
  CopyRight2 : Subsystem  Description=|  mask(Copyright Information){none=on}
      | Copyright info block.                                               
      |                                                                     
      | Place copyright information at the top of every subsystem in design.
      mask prompts: none "No parameters"
      mask help: Place copyright information at the top of every subsystem in design.
      mask Display:
      | NxtrConf = 'Nexteer Confidential';
      | 
      | sys = bdroot; %handle for the current model ("system")
      | first = get_param(sys,'Created');
      | first = first(end-3:end);  %year is last four digits
      | 
      | last = get_param(sys,'LastModifiedDate');
      | if isempty(last)
      |     last = datestr(now,'yyyy');
      | else
      |     last = last(end-3:end);
      | end
      | 
      | if strcmp(first,last)
      |     fprintf('%s -- Copyright %s Nexteer',NxtrConf,first)
      | else
      |     fprintf('%s -- %s%s- %s Nexteer',NxtrConf,char(169),first,last)
      | end
  Data Store Read1 : DataStoreRead  DataStoreName=RamBuf
  Data Store Read2 : DataStoreRead  DataStoreName=IgnCycSampleCntrAry
  Data Store Write1 : DataStoreWrite  DataStoreName=RamBuf
  Data Store Write6 : DataStoreWrite  DataStoreName=IgnCycSampleCntrAry
  Dont clear Nvm Data : Subsystem  TreatAsAtomicUnit=on
  For Iterator Subsystem : Subsystem  TreatAsAtomicUnit=on
  If : If  IfExpression=u1
  wires:
  Constant/1 -> For Iterator Subsystem/1("SigCnt ")
  If/2 -> Dont clear Nvm Data/Action
  If/1 -> Clear Nvm Data/Action
  TarSel_ArgIn/1 -> If/1
  Data Store Read1/1 -> Assignment1/1
  Assignment1/1 -> Data Store Write1/1
  Data Store Read2/1 -> Assignment4/1
  Constant4/1 -> Assignment4/2
  Assignment4/1 -> Data Store Write6/1
  Constant1/1 -> Assignment1/2

== system ES106A_StHlthSigStc/StHlthSigStc/ClrSigStcHlthData/ClrDataSample ==
  TarSel_ArgIn : Inport
  Action Port : ActionPort  ActionType=then
  Assignment1 : Assignment  IndexMode=Zero-based  IndexOptions=Assign all  Indices=1  OutputSizes=1
  Assignment4 : Assignment  IndexMode=Zero-based  IndexOptions=Assign all  Indices=1  OutputSizes=1
  Clear Nvm Data : Subsystem  TreatAsAtomicUnit=on
  Constant : Constant  Value=SIGCNT_ULS_U08
  Constant1 : Constant  Value=0  OutDataTypeStr=uint8
  Constant4 : Constant  Value=0  OutDataTypeStr=uint32
  CopyRight2 : Subsystem  Description=|  mask(Copyright Information){none=on}
      | Copyright info block.                                               
      |                                                                     
      | Place copyright information at the top of every subsystem in design.
      mask prompts: none "No parameters"
      mask help: Place copyright information at the top of every subsystem in design.
      mask Display:
      | NxtrConf = 'Nexteer Confidential';
      | 
      | sys = bdroot; %handle for the current model ("system")
      | first = get_param(sys,'Created');
      | first = first(end-3:end);  %year is last four digits
      | 
      | last = get_param(sys,'LastModifiedDate');
      | if isempty(last)
      |     last = datestr(now,'yyyy');
      | else
      |     last = last(end-3:end);
      | end
      | 
      | if strcmp(first,last)
      |     fprintf('%s -- Copyright %s Nexteer',NxtrConf,first)
      | else
      |     fprintf('%s -- %s%s- %s Nexteer',NxtrConf,char(169),first,last)
      | end
  Data Store Read1 : DataStoreRead  DataStoreName=RamBuf
  Data Store Read2 : DataStoreRead  DataStoreName=IgnCycSampleCntrAry
  Data Store Write1 : DataStoreWrite  DataStoreName=RamBuf
  Data Store Write6 : DataStoreWrite  DataStoreName=IgnCycSampleCntrAry
  Dont clear Nvm Data : Subsystem  TreatAsAtomicUnit=on
  For Iterator Subsystem : Subsystem  TreatAsAtomicUnit=on
  If : If  IfExpression=u1
  wires:
  TarSel_ArgIn/1 -> If/1
  If/1 -> Clear Nvm Data/Action
  If/2 -> Dont clear Nvm Data/Action
  Constant/1 -> For Iterator Subsystem/1("SigCnt ")
  Data Store Read1/1 -> Assignment1/1
  Assignment1/1 -> Data Store Write1/1
  Data Store Read2/1 -> Assignment4/1
  Constant4/1 -> Assignment4/2
  Assignment4/1 -> Data Store Write6/1
  Constant1/1 -> Assignment1/2

== system ES106A_StHlthSigStc/StHlthSigStc/ClrSigStcHlthData/CopyRight2 ==

== system ES106A_StHlthSigStc/StHlthSigStc/ClrSigStcHlthData/GetApplicationID ==
  note: This client server is used to get application id of state health signal which is currently being processed.
  Constant : Constant  Value=APPL10_CNT_U08
  CopyRight2 : Subsystem  Description=|  mask(Copyright Information){none=on}
      | Copyright info block.                                               
      |                                                                     
      | Place copyright information at the top of every subsystem in design.
      mask prompts: none "No parameters"
      mask help: Place copyright information at the top of every subsystem in design.
      mask Display:
      | NxtrConf = 'Nexteer Confidential';
      | 
      | sys = bdroot; %handle for the current model ("system")
      | first = get_param(sys,'Created');
      | first = first(end-3:end);  %year is last four digits
      | 
      | last = get_param(sys,'LastModifiedDate');
      | if isempty(last)
      |     last = datestr(now,'yyyy');
      | else
      |     last = last(end-3:end);
      | end
      | 
      | if strcmp(first,last)
      |     fprintf('%s -- Copyright %s Nexteer',NxtrConf,first)
      | else
      |     fprintf('%s -- %s%s- %s Nexteer',NxtrConf,char(169),first,last)
      | end
  ApplId : Outport
  wires:
  Constant/1 -> ApplId/1

== system ES106A_StHlthSigStc/StHlthSigStc/GetSigStcHlthData/CopyRight2 ==

== system ES106A_StHlthSigStc/StHlthSigStc/GetSigStcHlthData/If Action Subsystem ==
  Action Port : ActionPort  ActionType=else
  Constant : Constant  Value=ENOTOK_CNT_U08
  CopyRight2 : Subsystem  Description=|  mask(Copyright Information){none=on}
      | Copyright info block.                                               
      |                                                                     
      | Place copyright information at the top of every subsystem in design.
      mask prompts: none "No parameters"
      mask help: Place copyright information at the top of every subsystem in design.
      mask Display:
      | NxtrConf = 'Nexteer Confidential';
      | 
      | sys = bdroot; %handle for the current model ("system")
      | first = get_param(sys,'Created');
      | if(isempty(first))
      |     first = datestr(now,'yyyy');
      | else
      |     first = first(end-3:end);  %year is last four digits
      | end
      | 
      | last = get_param(sys,'LastModifiedDate');
      | if isempty(last)
      |     last = datestr(now,'yyyy');
      | else
      |     last = last(end-3:end);
      | end
      | 
      | if strcmp(first,last)
      |     fprintf('%s -- Copyright %s Nexteer',NxtrConf,first)
      | else
      |     fprintf('%s -- %s%s- %s Nexteer',NxtrConf,char(169),first,last)
      | end
  GetSigStcHlthData_StdRtn : Outport
  wires:
  Constant/1 -> GetSigStcHlthData_StdRtn/1

== system ES106A_StHlthSigStc/StHlthSigStc/GetSigStcHlthData/If Action Subsystem1 ==
  In1 : Inport
  Action Port : ActionPort  ActionType=then
  CopyRight2 : Subsystem  Description=|  mask(Copyright Information){none=on}
      | Copyright info block.                                               
      |                                                                     
      | Place copyright information at the top of every subsystem in design.
      mask prompts: none "No parameters"
      mask help: Place copyright information at the top of every subsystem in design.
      mask Display:
      | NxtrConf = 'Nexteer Confidential';
      | 
      | sys = bdroot; %handle for the current model ("system")
      | first = get_param(sys,'Created');
      | first = first(end-3:end);  %year is last four digits
      | 
      | last = get_param(sys,'LastModifiedDate');
      | if isempty(last)
      |     last = datestr(now,'yyyy');
      | else
      |     last = last(end-3:end);
      | end
      | 
      | if strcmp(first,last)
      |     fprintf('%s -- Copyright %s Nexteer',NxtrConf,first)
      | else
      |     fprintf('%s -- %s%s- %s Nexteer',NxtrConf,char(169),first,last)
      | end
  Data Store Read : DataStoreRead  DataStoreName=IgnCycSampleCntrAry
  GetSigStcHlthData : Subsystem
  If : If
  If Action Subsystem : Subsystem  TreatAsAtomicUnit=on
  Merge : Merge
  Selector : Selector  IndexMode=Zero-based  InputPortWidth=22  IndexOptions=Starting index (port)  Indices=[1 3]  OutputSizes=1
  BufPtr_ArgOut : Outport
  GetSigStcHlthData_StdRtn : Outport  Port=2
  wires:
  Data Store Read/1 -> Selector/1
  Selector/1 -> If/1
  If/1 -> GetSigStcHlthData/Action
  In1/1 -> GetSigStcHlthData/1(SigId_ArgIn), Selector/2
  If/2 -> If Action Subsystem/Action
  GetSigStcHlthData/2(GetSigStcHlthData_StdRtn) -> Merge/1
  If Action Subsystem/1(GetSigStcHlthData_StdRtn1) -> Merge/2
  Merge/1 -> GetSigStcHlthData_StdRtn/1
  GetSigStcHlthData/1(BufPtr_ArgOut) -> BufPtr_ArgOut/1
